simulink model "SIMULATOR_15_11"  (R2023b)
settings: Solver=VariableStepAuto  StartTime=0.0  StopTime=20  RelTol=1e-3
values from neighbouring files (symbols this model uses):
  a = [ 0 0 1 1 ... (first row only)    [GeoGebraModel.m]    (also in main.m)
  b = [-0.075 -0.075  0.075 0.075 ... (first row only)    [GeoGebraModel.m]    (also in main.m = [-0.075 -0.075  0.075  0.075)
  f_level = 2    [main.m]
  f_max = 100    [main.m]
  f_min = 10    [main.m]
  Iz = 1/12*m*(l^2+b^2)    (= 0.000141145833333)    [main.m]
  K_d = diag([2 80 1])    [main.m]
  K_i = diag([15 15 1])    [main.m]
  K_p = diag([10 10 1])    [main.m]
  m = 4    [InverseKinematicsWrenchMatrix.m]    (also in Kernel_translation.m = length(A); WrenchMatrix.m; constraintGradient.m; main.m = 0.1355)
  Wp = m*[0 -g 0]'    [main.m]
  y_0 = [.25 .5 0]'    [main.m]
  y_reference = [x_ref y_ref phi_ref]'    [main.m]
settings Model: Creator=eliasoa  LastModifiedBy=eliasoa

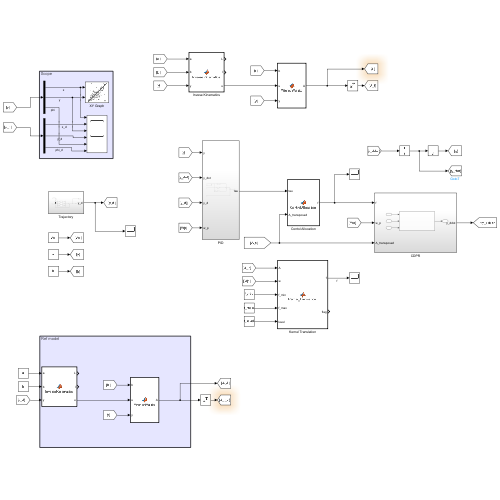
[thumbnail: Simulink's stored preview of the top-level diagram]
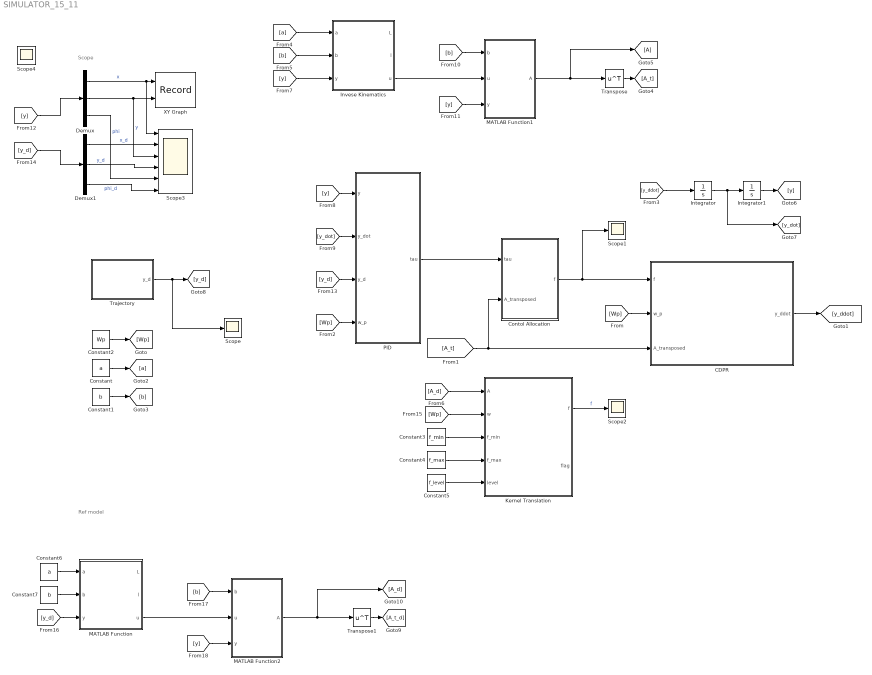
== system SIMULATOR_15_11 ==
  note: Ref model
  note: Scope
  CDPR : Subsystem
  Constant : Constant  Value=a
  Constant1 : Constant  Value=b
  Constant2 : Constant  Value=Wp
  Constant3 : Constant  Value=f_min
  Constant4 : Constant  Value=f_max
  Constant5 : Constant  Value=f_level
  Constant6 : Constant  Value=a
  Constant7 : Constant  Value=b
  Contol Allocation : MATLAB Function  TreatAsAtomicUnit=on
  Demux : Demux  Outputs=3
  Demux1 : Demux  Outputs=3
  Goto5 : Goto
  Integrator : Integrator  InitialCondition=[0; 0; 0];
  Integrator1 : Integrator  InitialCondition=y_0
  Invese Kinematics : MATLAB Function  TreatAsAtomicUnit=on
  Kernel Translation : MATLAB Function  TreatAsAtomicUnit=on
  MATLAB Function : MATLAB Function  TreatAsAtomicUnit=on
  MATLAB Function1 : MATLAB Function  TreatAsAtomicUnit=on
  MATLAB Function2 : MATLAB Function  TreatAsAtomicUnit=on
  "PID " : Subsystem
  Scope{,1..2,4} (4 alike) : Scope
  Scope3 : Scope  NumInputPorts=6
  Trajectory : Subsystem
  Transpose : Math  Operator=transpose
  Transpose1 : Math  Operator=transpose
  XY Graph : Record  FileSettingsInternal="{\"entries\":[{\"content\":{\"excelSettings\":{\"content\":{},\"type\":\"Streamout.ExcelSettings\"}},\"type\":\"Streamout.FileSettingStorage\",\"uuid\":\"\"}],\"packageUris\":[\"http:\\/\\/schema.mathworks.com\\/mf0\\/streamout_blocks\\/R2020a\"],\"version\":\"1.0\"}"  Layout=[1 1]  SignalsInternal="{\"entries\":[{\"content\":{\"signals\":[{\"content\":{\"blockPath\":[],\"dimensions\":[1,1],\"domain\":\"\",\"lineColor\":\"#4dbeee\",\"plots\":[1],\"port\":1,\"sid\":[\"\"],\"signalID\":1980,\"signalName\":\"x\"},\"type\":\"RecordBlkView.Signal\",\"uuid\":\"\"},{\"content\":{\"blockPath\":[],\"dimensions\":[1,1],\"domain\":\"\",\"lineColor\":\"#a2142f\",\"plots\":[1],\"port\":2,\"sid\":[\"\"],\"signalID\":1984,\"signalName\":\"y\"},\"type\":\"RecordBlkView.Signal\",\"uuid\":\"\"}]},\"type\":\"RecordBlkView.InputSignals\",\"uuid\":\"\"}],\"packageUris\":[\"http:\\/\\/schema.mathworks.com\\/mf0\\/streamout_blocks\\/R2020a\"],\"version\":\"1.0\"}"  VisualizationBindings="{\"xyplotplugin\":{\"info\":[{\"series\":[{\"bindingParametersList\":[{\"parameter\":\"X-Axis\",\"signalID\":1980,\"signalName\":\"x\"},{\"parameter\":\"Y-Axis\",\"signalID\":1984,\"signalName\":\"y\"}],\"seriesID\":8614}],\"subplotID\":1}]}}"  CompatibilityTag=XY
  wires:
  "PID "/1(tau) -> Contol Allocation/1(tau)
  Contol Allocation/1(f) -> CDPR/1(f), Scope1/1
  [A_t] -> CDPR/3(A_transposed), Contol Allocation/2(A_transposed)
  Integrator/1 -> [y_dot], Integrator1/1
  CDPR/1(y_ddot) -> [y_ddot]
  Constant2/1 -> [Wp]
  [Wp] -> CDPR/2(w_p)
  [Wp] -> "PID "/4(w_p)
  [y_ddot] -> Integrator/1
  Constant1/1 -> [b]
  Constant/1 -> [a]
  [b] -> Invese Kinematics/2(b)
  [a] -> Invese Kinematics/1(a)
  MATLAB Function1/1(A) -> Goto5/1, Transpose/1
  Transpose/1 -> [A_t]
  Invese Kinematics/3(u) -> MATLAB Function1/2(u)
  [y] -> Invese Kinematics/3(y)
  Integrator1/1 -> [y]
  [y] -> "PID "/1(y)
  [y_dot] -> "PID "/2(y_dot)
  [b] -> MATLAB Function1/1(b)
  [y] -> MATLAB Function1/3(y)
  [y_d] -> "PID "/3(y_d)
  Trajectory/1(y_d) -> Scope/1, [y_d]
  Constant5/1 -> Kernel Translation/5(level)
  Constant4/1 -> Kernel Translation/4(f_max)
  Constant3/1 -> Kernel Translation/3(f_min)
  [A_d] -> Kernel Translation/1(A)
  [Wp] -> Kernel Translation/2(w)
  Kernel Translation/1(f) -> Scope2/1  "f"
  Demux1/3 -> Scope3/6  "phi_d"
  Demux1/2 -> Scope3/4  "y_d"
  Demux1/1 -> Scope3/2  "x_d"
  Demux/3 -> Scope3/5  "phi"
  Demux/2 -> XY Graph/2, Scope3/3  "y"
  Demux/1 -> Scope3/1, XY Graph/1  "x"
  [y] -> Demux/1
  [y_d] -> Demux1/1
  Constant7/1 -> MATLAB Function/2(b)
  Constant6/1 -> MATLAB Function/1(a)
  [y_d] -> MATLAB Function/3(y)
  [y] -> MATLAB Function2/3(y)
  MATLAB Function/3(u) -> MATLAB Function2/2(u)
  [b] -> MATLAB Function2/1(b)
  MATLAB Function2/1(A) -> [A_d], Transpose1/1
  Transpose1/1 -> [A_t_d]

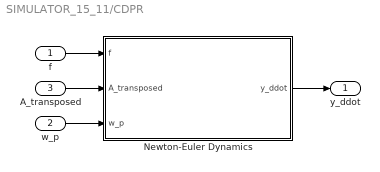
== system SIMULATOR_15_11/CDPR ==
  f : Inport
  w_p : Inport  Port=2
  A_transposed : Inport  Port=3
  "Newton-Euler Dynamics " : Subsystem
  y_ddot : Outport
  wires:
  "Newton-Euler Dynamics "/1(y_ddot) -> y_ddot/1
  A_transposed/1 -> "Newton-Euler Dynamics "/2(A_transposed)
  f/1 -> "Newton-Euler Dynamics "/1(f)
  w_p/1 -> "Newton-Euler Dynamics "/3(w_p)

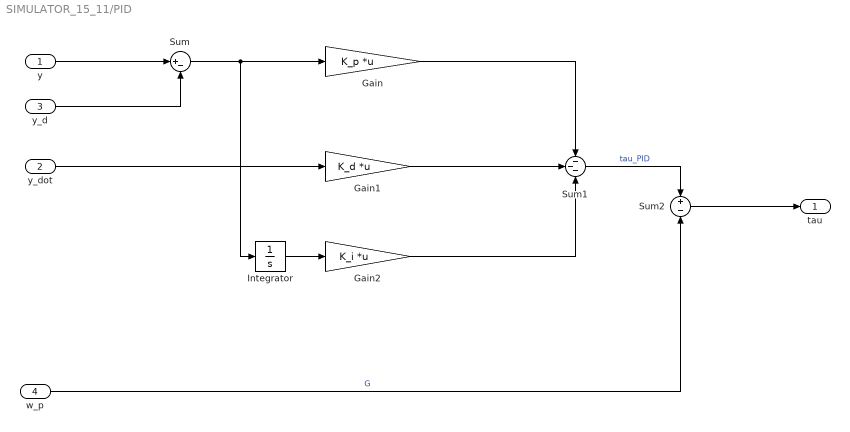
== system SIMULATOR_15_11/PID  ==
  y : Inport
  y_dot : Inport  Port=2
  y_d : Inport  Port=3
  w_p : Inport  Port=4
  Gain : Gain  Gain=K_p  Multiplication=Matrix(K*u)
  Gain1 : Gain  Gain=K_d  Multiplication=Matrix(K*u)
  Gain2 : Gain  Gain=K_i  Multiplication=Matrix(K*u)
  Integrator : Integrator
  Sum : Sum  Inputs=|+-
  Sum1 : Sum  Inputs=---
  Sum2 : Sum  Inputs=+|-
  tau : Outport
  wires:
  y/1 -> Sum/1
  y_d/1 -> Sum/2
  Sum/1 -> Integrator/1, Gain/1
  y_dot/1 -> Gain1/1
  Sum2/1 -> tau/1
  w_p/1 -> Sum2/2  "G"
  Gain1/1 -> Sum1/2
  Gain/1 -> Sum1/1
  Integrator/1 -> Gain2/1
  Gain2/1 -> Sum1/3
  Sum1/1 -> Sum2/1  "tau_PID"

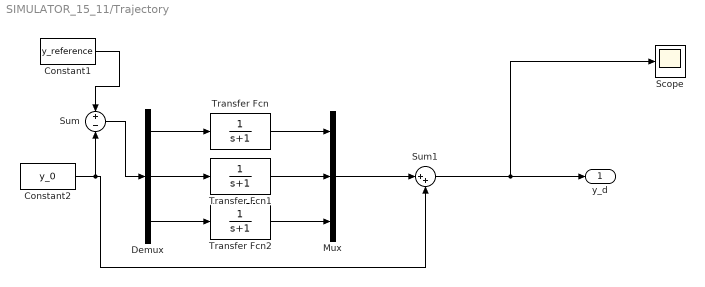
== system SIMULATOR_15_11/Trajectory ==
  Constant1 : Constant  Value=y_reference
  Constant2 : Constant  Value=y_0
  Demux : Demux  Outputs=3
  Mux : Mux  Inputs=3
  Scope : Scope
  Sum : Sum  Inputs=+-
  Sum1 : Sum  Inputs=|++
  Transfer Fcn : TransferFcn  Denominator=[1 1]
  Transfer Fcn1 : TransferFcn  Denominator=[1 1]
  Transfer Fcn2 : TransferFcn  Denominator=[1 1]
  y_d : Outport
  wires:
  Transfer Fcn2/1 -> Mux/3
  Transfer Fcn1/1 -> Mux/2
  Transfer Fcn/1 -> Mux/1
  Demux/2 -> Transfer Fcn1/1
  Demux/1 -> Transfer Fcn/1
  Demux/3 -> Transfer Fcn2/1
  Constant1/1 -> Sum/1
  Mux/1 -> Sum1/1
  Sum1/1 -> y_d/1, Scope/1
  Sum/1 -> Demux/1
  Constant2/1 -> Sum1/2, Sum/2

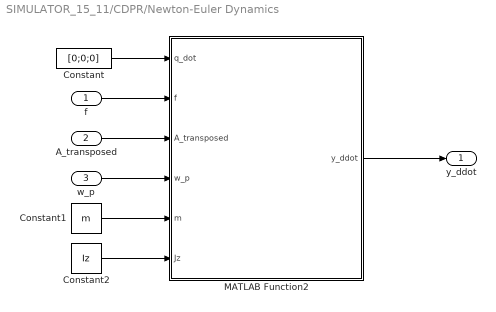
== system SIMULATOR_15_11/CDPR/Newton-Euler Dynamics  ==
  f : Inport
  A_transposed : Inport  Port=2
  w_p : Inport  Port=3
  Constant : Constant  Value=[0;0;0]
  Constant1 : Constant  Value=m
  Constant2 : Constant  Value=Iz
  MATLAB Function2 : MATLAB Function  TreatAsAtomicUnit=on
  y_ddot : Outport
  wires:
  MATLAB Function2/1(y_ddot) -> y_ddot/1
  f/1 -> MATLAB Function2/2(f)
  Constant/1 -> MATLAB Function2/1(q_dot)
  A_transposed/1 -> MATLAB Function2/3(A_transposed)
  Constant1/1 -> MATLAB Function2/5(m)
  Constant2/1 -> MATLAB Function2/6(Jz)
  w_p/1 -> MATLAB Function2/4(w_p)

== matlab function SIMULATOR_15_11/MATLAB Function1 ==
  data: b input; u input; A output; y input
function A = WrenchMatrix(b, u, y)
    A = WrenchMatrix(b, u, y);
end

== matlab function SIMULATOR_15_11/Invese Kinematics ==
  data: a input; L output; b input; y input; l output; u output
function [L,l,u] = InverseKinematics(a, b, y)
    [L,l,u] = InverseKinematics(a, b, y);
end

== matlab function SIMULATOR_15_11/MATLAB Function ==
  data: a input; L output; b input; y input; l output; u output
function [L,l,u] = InverseKinematics(a, b, y)
    [L,l,u] = InverseKinematics(a, b, y);
end

== matlab function SIMULATOR_15_11/Contol Allocation ==
  data: tau input; f output; A_transposed input
function f = ControlAllocation(tau, A_transposed)
A_PseudoInv = A_transposed'/(A_transposed*A_transposed');
f = A_PseudoInv*tau;
end

== matlab function SIMULATOR_15_11/CDPR/Newton-Euler Dynamics /MATLAB Function2 ==
  data: q_dot input; y_ddot output; f input; A_transposed input; w_p input; m input; Jz input
function y_ddot = NewtonEuler_Dynamics(q_dot, f, A_transposed, w_p, m, Jz)

y_ddot = CDPR_NewtonEuler_Dynamics(q_dot, f, A_transposed, w_p, m, Jz);

== matlab function SIMULATOR_15_11/Kernel Translation ==
  data: A input; f output; w input; f_min input; f_max input; level input; flag output
function [f, flag] = Kernel_translation(A,w,f_min,f_max,level)
[f, flag] = Kernel_translation(A,w,f_min,f_max,level);
end

== matlab function SIMULATOR_15_11/MATLAB Function2 ==
  data: b input; u input; A output; y input
function A = WrenchMatrix(b, u, y)
    A = WrenchMatrix(b, u, y);
end
